simulink model "Faultsimulation"  (R2021a)
settings: Solver=VariableStepAuto  StartTime=0.0  StopTime=10.0  MaxStep=1e-4  RelTol=1e-3  EnableMultiTasking=on
undefined symbols (not defined in the file or in its folder): D1, Delta
libraries: spsSeriesRLCBranchLib x6, spsThreePhaseVIMeasurementLib x4, spsThreePhaseBreakerLib x4, spsCurrentMeasurementLib x2, spsFourierLib x2, spsThreePhaseParallelRLCLoadLib x1, spsThreePhaseTransformerTwoWindingsLib x1, spsThreePhaseFaultLib x1, spsSynchronousMachinepuStandardLib x1, spsThreePhaseProgrammableVoltageSourceLib x1, spspowerguiLib x1
settings Model: Creator=ASUS  LastModifiedBy=Maruf
settings SolverCC: AlgebraicLoopSolver=TrustRegion
settings DataIOCC: ReturnWorkspaceOutputs=off
settings OptimizationCC: LifeSpan=inf
settings DebuggingCC: SFMachineParentedDataDiag=warning  ArithmeticOperatorsInVariantConditions=warning
settings SFSimCC: SimUseLocalCustomCode=off  CustomCodeUndefinedFunction=UseInterfaceOnly
settings RTWCC: RTWUseLocalCustomCode=off
settings CodeAppCC: StateflowObjectComments=on
settings SimscapeCC: SimscapeNormalizeSystem=off

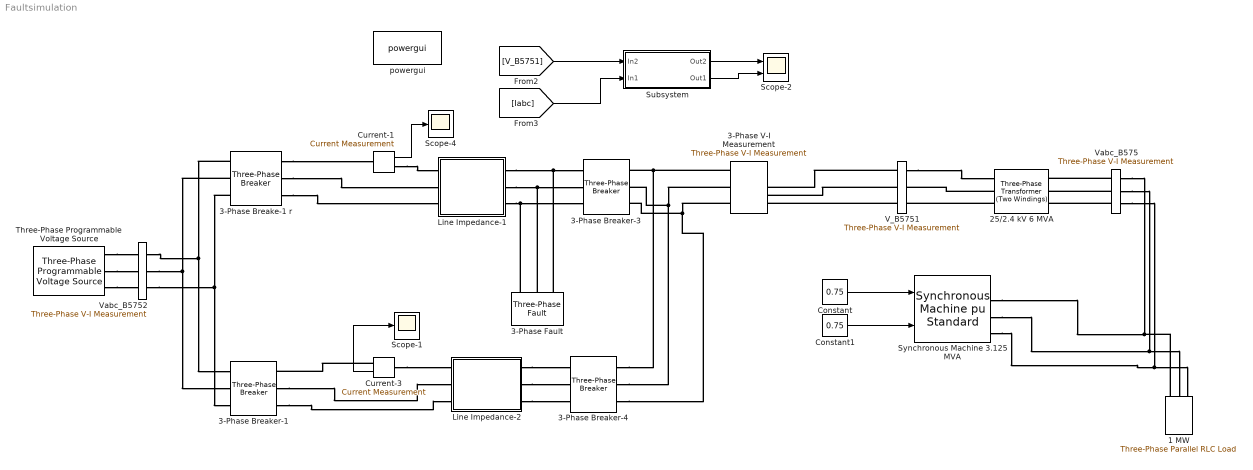
== system Faultsimulation ==
  1 MW : spsThreePhaseParallelRLCLoadLib/Three-Phase Parallel RLC Load  LConnTagsString=A|B|C  Configuration=Y (grounded)  NominalVoltage=2400  Vabc=[1e3 1e3 1e3]  Vabcp=[1e3 1e3 1e3]  NominalFrequency=60  UnbalancedPower=off  ActivePower=1e6  InductivePower=0  CapacitivePower=0  Pabc=[10e3 9e3 11e3]  QLabc=[100 90 110]  QCabc=[100 90 110]  Pabcp=[10e3 9e3 11e3]  QLabcp=[100 90 110]  QCabcp=[100 90 110]  Measurements=None  LoadType=constant Z
  25/2.4 kV 6 MVA : spsThreePhaseTransformerTwoWindingsLib/Three-Phase Transformer (Two Windings)  Winding1Connection=Yg  Winding2Connection=Delta (D1)  CoreType=Three single-phase transformers  SetSaturation=off  Hysteresis=off  DataFile='hysteresis'  SetInitialFlux=off  Measurements=None  UNITS=pu  NominalPower=[6e6 , 60 ]  Winding1=[25e3 , 0.0015 , 0.03 ]  Winding2=[2.4e3 , 0.0015 , 0.03 ]  Rm=200  Lm=200  L0=0.5  Saturation=[ 0,0 ; 0.0024,1.2 ; 1.0,1.52 ]  InitialFluxes=[ 0.8 , -0.8 , 0.7 ]  BreakLoop=off  DiscreteSolver=Trapezoidal iterative  DataType=off  TransfoNumber=1
  3-Phase V-I Measurement : spsThreePhaseVIMeasurementLib/Three-Phase V-I Measurement  VoltageMeasurement=phase-to-ground  SetLabelV=off  LabelV=B25kV  Vpu=on  VpuLL=off  CurrentMeasurement=yes  SetLabelI=off  LabelI=Iabc  Ipu=off  Pbase=100e6  Vbase=25e3  OutputType=Complex  PhasorSimulation=off  PSBequivalent=0
  3-Phase Breake-1 r : spsThreePhaseBreakerLib/Three-Phase Breaker  InitialState=closed  SwitchA=on  SwitchB=on  SwitchC=on  SwitchTimes=[3.4 4.4]  External=off  BreakerResistance=0.01  SnubberResistance=1e6  SnubberCapacitance=inf  Measurements=Breaker voltages and currents
  3-Phase Breaker-1 : spsThreePhaseBreakerLib/Three-Phase Breaker  InitialState=closed  SwitchA=on  SwitchB=on  SwitchC=on  SwitchTimes=[13.2 14.2]  External=off  BreakerResistance=0.01  SnubberResistance=1e6  SnubberCapacitance=inf  Measurements=Breaker voltages and currents
  3-Phase Breaker-3 : spsThreePhaseBreakerLib/Three-Phase Breaker  InitialState=closed  SwitchA=on  SwitchB=on  SwitchC=on  SwitchTimes=[3.4 4.4]  External=off  BreakerResistance=0.01  SnubberResistance=1e6  SnubberCapacitance=inf  Measurements=Breaker voltages and currents
  3-Phase Breaker-4 : spsThreePhaseBreakerLib/Three-Phase Breaker  InitialState=closed  SwitchA=on  SwitchB=on  SwitchC=on  SwitchTimes=[13.2 14.2]  External=off  BreakerResistance=0.01  SnubberResistance=1e6  SnubberCapacitance=inf  Measurements=Breaker voltages and currents
  3-Phase Fault : spsThreePhaseFaultLib/Three-Phase Fault  InitialStates=0  FaultA=on  FaultB=on  FaultC=on  GroundFault=on  SwitchTimes=[3.3 4.3]  External=off  SwitchStatus=NaN  FaultResistance=0.01  GroundResistance=0.001  SnubberResistance=1e6  SnubberCapacitance=inf  Measurements=Fault currents
  Constant : Constant  Value=0.75
  Constant1 : Constant  Value=0.75
  Current-1 : spsCurrentMeasurementLib/Current Measurement  PhasorSimulation=off  OutputType=Complex  PSBequivalent=0
  Current-3 : spsCurrentMeasurementLib/Current Measurement  PhasorSimulation=off  OutputType=Complex  PSBequivalent=0
  Line Impedance-1 : Subsystem
  Line Impedance-2 : Subsystem
  Scope-1 : Scope
  Scope-2 : Scope  NumInputPorts=2
  Scope-4 : Scope
  Subsystem : Subsystem
  Synchronous Machine 3.125 MVA : spsSynchronousMachinepuStandardLib/Synchronous Machine pu Standard  PresetModel=No  MechanicalLoad=Mechanical power Pm  ShowDetailedParameters=on  RotorType=Salient-pole  Units=per unit standard parameters  MeasurementBus=off  NominalParameters=[3.125e6 2400 60]  Reactances1=[ 1.81, 0.3, 0.23, 1.76, 0.65, 0.25, 0.15 ]  Reactances2=[1.56, 0.296, 0.177, 1.06, 0.177, 0.052]  dAxisTimeConstants=Short-circuit  qAxisTimeConstants=Open-circuit  TimeConstants1="[ 4.4849  0.0681  0.1  ]"  TimeConstants2=[ 8.0, 0.03, 1.0, 0.07 ]  TimeConstants3="[  4.49  0.0681  0.0513  ]"  TimeConstants4=[ 8.0, 0.03, 0.3371, 0.0295 ]  TimeConstants5=[ 3.7, 0.05, 0.05 ]  TimeConstants6=[ 1.3201, 0.023, 1.0, 0.07 ]  TimeConstants7=[0.012 0.003 0.003]  TimeConstants8=[ 1.3201, 0.0231, 0.3371, 0.0295 ]  StatorResistance=0.0036  Mechanical=[1.07 0 2]  PolePairs=20  InitialConditions="[ 0  0  0  0  0  0  0  0  1 ]"  SetSaturation=off  Saturation=[0.6404,0.7127,0.8441,0.9214,0.9956,1.082,1.19,1.316,1.457;0.7,0.7698,0.8872,0.9466,0.9969,1.046,1.1,1.151,1.201]  LoadFlowParameters=[1,0,0,0,0]  TsPowergui=0  TsBlock=-1  IterativeModel=Trapezoidal non iterative  IterativeDiscreteModel=Trapezoidal non iterative  BusType=PV  Pref=0  Qref=0  Qmin=-inf  Qmax=inf  PLF=0  QLF=0
      settings: SourceProductBaseCode=PS
  Three-Phase Programmable Voltage Source : spsThreePhaseProgrammableVoltageSourceLib/Three-Phase Programmable Voltage Source  PositiveSequence="[25e3  0 60]"  VariationEntity=None  VariationType=Table of time-amplitude pairs  VariationTypeAlt=Step  VariationStep=0.5  VariationRate=10  VariationMagnitude=0.3  VariationFrequency=2  VariationTiming=[1 2]  VariationPhaseA=off  Amplitudes=[1 0.8 1.2 1.0]  TimeValues=[0 0.1 0.15 0.2]  HarmonicGeneration=off  HarmonicA=[3 0.2 -25 0]  HarmonicB=[2 0.15 35 2]  Timing="[0.05  3]"  BusType=swing  Pref=0  Qref=0  Qmin=-inf  Qmax=inf
  V_B5751 : spsThreePhaseVIMeasurementLib/Three-Phase V-I Measurement  VoltageMeasurement=phase-to-ground  SetLabelV=on  LabelV=V_B5751  Vpu=on  VpuLL=off  CurrentMeasurement=yes  SetLabelI=on  LabelI=Iabc  Ipu=off  Pbase=100e6  Vbase=25e3  OutputType=Complex  PhasorSimulation=off  PSBequivalent=0
  Vabc_B575 : spsThreePhaseVIMeasurementLib/Three-Phase V-I Measurement  VoltageMeasurement=phase-to-ground  SetLabelV=on  LabelV=Vabc_B575  Vpu=on  VpuLL=off  CurrentMeasurement=no  SetLabelI=off  LabelI=Iabc  Ipu=off  Pbase=100e6  Vbase=2.4e3  OutputType=Complex  PhasorSimulation=off  PSBequivalent=0
  Vabc_B5752 : spsThreePhaseVIMeasurementLib/Three-Phase V-I Measurement  VoltageMeasurement=phase-to-ground  SetLabelV=on  LabelV=Vabc_B5752  Vpu=on  VpuLL=off  CurrentMeasurement=no  SetLabelI=off  LabelI=Iabc  Ipu=off  Pbase=100e6  Vbase=25e3  OutputType=Complex  PhasorSimulation=off  PSBequivalent=0
  powergui : spspowerguiLib/powergui  Priority=1  SimulationMode=Discrete  SampleTime=5e-5  frequency=60  Iterations=50  frequencyindice=60  Pbase=100e6  ErrMax=1e-4  UnitsV=kV  UnitsW=MW  buscounter=0  FunctionMessages=off  echomessages=off  EnableUseOfTLC=off  CurrentSourceSwitches=off  DisableSnubberDevices=off  DisableRonSwitches=off  DisableVfSwitches=off  DisplayEquations=off  AutomaticDiscreteSolvers=off  SolverType=Tustin/Backward Euler (TBE)  Interpol=off  ExternalGateDelay=off  methode=off  Ts=100  x0status=blocks  SPID=on  SwTol=0  HookPort=off  NonlinearTolerance=1e-4  nMaxIteration=100  ContinueOnMaxIteration=off  RestoreLinks=warning  ResistiveCurrentMeasurement=off  Frange=[0:2:500]  Ylog=off  Xlog=on  ShowGrid=off  save=off  variable=ZData  structure=0  ZoomFFT=off  StartTime=0.0  cycles=1  DisplayStyle=1  fundamental=60  FreqAxis=off  MaxFrequency=1000  frequencyindicesteady=1  RmsSteady=1  display=off
  wires:
  Current-1/1 -> Scope-4/1
  Current-3/1 -> Scope-1/1
  Constant/1 -> Synchronous Machine 3.125 MVA/1
  Constant1/1 -> Synchronous Machine 3.125 MVA/2
  [V_B5751] -> Subsystem/1(In2)
  Subsystem/1(Out2) -> Scope-2/1
  [Iabc] -> Subsystem/2(In1)
  Subsystem/2(Out1) -> Scope-2/2
  connections:
  Three-Phase Programmable Voltage Source/RConn1 -- Vabc_B5752/LConn1
  Three-Phase Programmable Voltage Source/RConn2 -- Vabc_B5752/LConn2
  Three-Phase Programmable Voltage Source/RConn3 -- Vabc_B5752/LConn3
  3-Phase Breake-1 r/LConn1 -- Vabc_B5752/RConn1 -- 3-Phase Breaker-1/LConn1
  3-Phase Breake-1 r/LConn2 -- 3-Phase Breaker-1/LConn2 -- Vabc_B5752/RConn2
  3-Phase Breake-1 r/LConn3 -- Vabc_B5752/RConn3 -- 3-Phase Breaker-1/LConn3
  3-Phase Breake-1 r/RConn1 -- Current-1/LConn1
  3-Phase Breake-1 r/RConn2 -- Line Impedance-1/LConn2
  3-Phase Breake-1 r/RConn3 -- Line Impedance-1/LConn3
  Current-1/RConn1 -- Line Impedance-1/LConn1
  Current-3/RConn1 -- 3-Phase Breaker-1/RConn1
  Current-3/LConn1 -- Line Impedance-2/LConn1
  3-Phase Breaker-1/RConn2 -- Line Impedance-2/LConn2
  3-Phase Breaker-1/RConn3 -- Line Impedance-2/LConn3
  Line Impedance-1/RConn1 -- 3-Phase Fault/LConn1 -- 3-Phase Breaker-3/LConn1
  Line Impedance-1/RConn2 -- 3-Phase Fault/LConn2 -- 3-Phase Breaker-3/LConn2
  Line Impedance-1/RConn3 -- 3-Phase Fault/LConn3 -- 3-Phase Breaker-3/LConn3
  Line Impedance-2/RConn1 -- 3-Phase Breaker-4/LConn1
  Line Impedance-2/RConn2 -- 3-Phase Breaker-4/LConn2
  Line Impedance-2/RConn3 -- 3-Phase Breaker-4/LConn3
  3-Phase V-I Measurement/LConn2 -- 3-Phase Breaker-4/RConn2 -- 3-Phase Breaker-3/RConn2
  3-Phase Breaker-4/RConn1 -- 3-Phase V-I Measurement/LConn1 -- 3-Phase Breaker-3/RConn1
  3-Phase V-I Measurement/LConn3 -- 3-Phase Breaker-4/RConn3 -- 3-Phase Breaker-3/RConn3
  V_B5751/LConn3 -- 3-Phase V-I Measurement/RConn3
  25/2.4 kV 6 MVA/LConn2 -- V_B5751/RConn2
  25/2.4 kV 6 MVA/LConn3 -- V_B5751/RConn3
  Vabc_B575/LConn1 -- 25/2.4 kV 6 MVA/RConn1
  Vabc_B575/LConn2 -- 25/2.4 kV 6 MVA/RConn2
  Vabc_B575/LConn3 -- 25/2.4 kV 6 MVA/RConn3
  Synchronous Machine 3.125 MVA/RConn2 -- Vabc_B575/RConn2 -- 1 MW/LConn2
  Synchronous Machine 3.125 MVA/RConn1 -- 1 MW/LConn1 -- Vabc_B575/RConn1
  V_B5751/LConn2 -- 3-Phase V-I Measurement/RConn2
  V_B5751/RConn1 -- 25/2.4 kV 6 MVA/LConn1
  V_B5751/LConn1 -- 3-Phase V-I Measurement/RConn1
  Synchronous Machine 3.125 MVA/RConn3 -- Vabc_B575/RConn3 -- 1 MW/LConn3

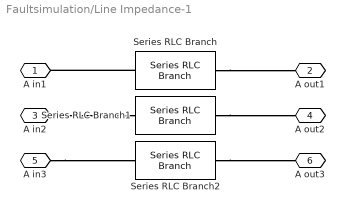
== system Faultsimulation/Line Impedance-1 ==
  Series RLC Branch : spsSeriesRLCBranchLib/Series RLC Branch  LConnTagsString=__new0  RConnTagsString=__new0  BranchType=RL  Resistance=2.92e-2  Inductance=2.82e-2  SetiL0=off  InitialCurrent=0  Capacitance=1e-6  Setx0=off  InitialVoltage=0  Measurements=None
  Series RLC Branch1 : spsSeriesRLCBranchLib/Series RLC Branch  LConnTagsString=__new0  RConnTagsString=__new0  BranchType=RL  Resistance=2.92e-2  Inductance=2.82e-2  SetiL0=off  InitialCurrent=0  Capacitance=1e-6  Setx0=off  InitialVoltage=0  Measurements=None
  Series RLC Branch2 : spsSeriesRLCBranchLib/Series RLC Branch  LConnTagsString=__new0  RConnTagsString=__new0  BranchType=RL  Resistance=2.92e-2  Inductance=2.82e-2  SetiL0=off  InitialCurrent=0  Capacitance=1e-6  Setx0=off  InitialVoltage=0  Measurements=None
  A in1 : PMIOPort  Side=Left
  A out1 : PMIOPort  Port=2  Side=Right
  A in2 : PMIOPort  Port=3  Side=Left
  A out2 : PMIOPort  Port=4  Side=Right
  A in3 : PMIOPort  Port=5  Side=Left
  A out3 : PMIOPort  Port=6  Side=Right
  connections:
  Series RLC Branch2/RConn1 -- A out3/RConn1
  Series RLC Branch1/RConn1 -- A out2/RConn1
  Series RLC Branch/RConn1 -- A out1/RConn1
  Series RLC Branch/LConn1 -- A in1/RConn1
  A in2/RConn1 -- Series RLC Branch1/LConn1
  A in3/RConn1 -- Series RLC Branch2/LConn1

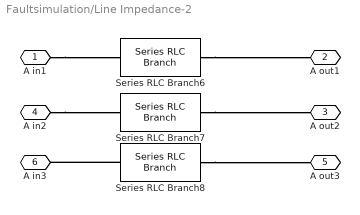
== system Faultsimulation/Line Impedance-2 ==
  Series RLC Branch6 : spsSeriesRLCBranchLib/Series RLC Branch  LConnTagsString=__new0  RConnTagsString=__new0  BranchType=RL  Resistance=2.92e-2  Inductance=2.82e-2  SetiL0=off  InitialCurrent=0  Capacitance=1e-6  Setx0=off  InitialVoltage=0  Measurements=None
  Series RLC Branch7 : spsSeriesRLCBranchLib/Series RLC Branch  LConnTagsString=__new0  RConnTagsString=__new0  BranchType=RL  Resistance=2.92e-2  Inductance=2.82e-2  SetiL0=off  InitialCurrent=0  Capacitance=1e-6  Setx0=off  InitialVoltage=0  Measurements=None
  Series RLC Branch8 : spsSeriesRLCBranchLib/Series RLC Branch  LConnTagsString=__new0  RConnTagsString=__new0  BranchType=RL  Resistance=2.92e-2  Inductance=2.82e-2  SetiL0=off  InitialCurrent=0  Capacitance=1e-6  Setx0=off  InitialVoltage=0  Measurements=None
  A in1 : PMIOPort  Side=Left
  A out1 : PMIOPort  Port=2  Side=Right
  A out2 : PMIOPort  Port=3  Side=Right
  "A in2 " : PMIOPort  Port=4  Side=Left
  A out3 : PMIOPort  Port=5  Side=Right
  A in3 : PMIOPort  Port=6  Side=Left
  connections:
  Series RLC Branch6/RConn1 -- A out1/RConn1
  Series RLC Branch8/LConn1 -- A in3/RConn1
  Series RLC Branch8/RConn1 -- A out3/RConn1
  Series RLC Branch7/RConn1 -- A out2/RConn1
  A in1/RConn1 -- Series RLC Branch6/LConn1
  "A in2 "/RConn1 -- Series RLC Branch7/LConn1

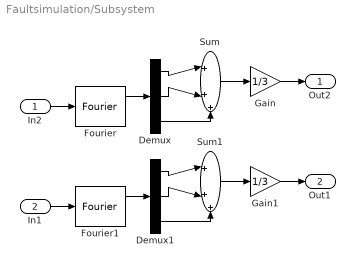
== system Faultsimulation/Subsystem ==
  In2 : Inport
  In1 : Inport  Port=2
  Demux : Demux  Outputs=3
  Demux1 : Demux  Outputs=3
  Fourier : spsFourierLib/Fourier  Freq=60  n=1  InInit=[0, 0]  Ts=50e-6
      settings: SourceProductBaseCode=PS
  Fourier1 : spsFourierLib/Fourier  Freq=60  n=1  InInit=[0, 0]  Ts=50e-6
      settings: SourceProductBaseCode=PS
  Gain : Gain  Gain=1/3
  Gain1 : Gain  Gain=1/3
  Sum : Sum  Inputs=|+++
  Sum1 : Sum  Inputs=|+++
  Out2 : Outport
  Out1 : Outport  Port=2
  wires:
  In2/1 -> Fourier/1
  Fourier/1 -> Demux/1
  Gain/1 -> Out2/1
  Demux/3 -> Sum/3
  Demux/2 -> Sum/2
  Sum/1 -> Gain/1
  Demux/1 -> Sum/1
  Demux1/1 -> Sum1/1
  Demux1/3 -> Sum1/3
  Fourier1/1 -> Demux1/1
  Gain1/1 -> Out1/1
  Sum1/1 -> Gain1/1
  In1/1 -> Fourier1/1
  Demux1/2 -> Sum1/2
